simulink model "OM1"  (R2018b)
settings: Solver=VariableStepAuto  StartTime=0.0  StopTime=t_final  MaxStep=0.001  RelTol=1e-3
undefined symbols (not defined in the file): K1, K2, Ki, Kia, Kp, Kpa, st, T0, T1, T2, Tzap
settings Model: Creator=Anton Mayorov  LastModifiedBy=bedla
settings SFSimCC: SimUseLocalCustomCode=off
settings RTWCC: RTWUseLocalCustomCode=off

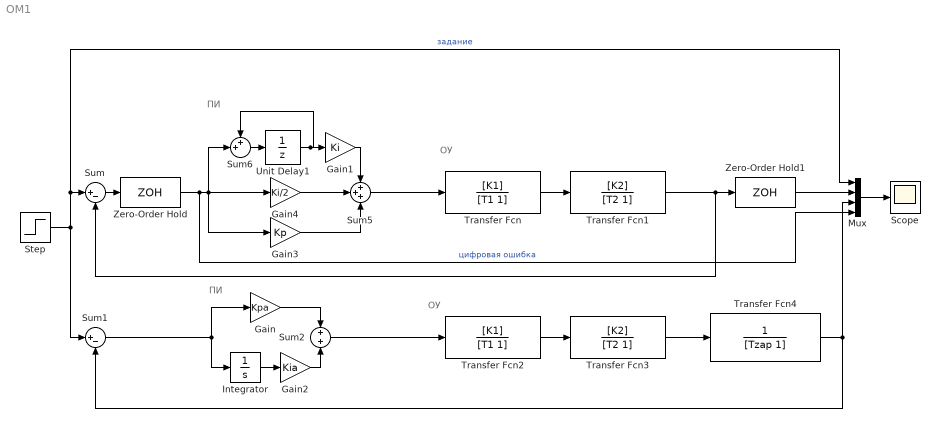
== system OM1 ==
  note: ПИ
  note: ПИ
  note: ОУ
  note: ОУ
  Gain : Gain  Gain=Kpa
  Gain1 : Gain  Gain=Ki
  Gain2 : Gain  Gain=Kia
  Gain3 : Gain  Gain=Kp
  Gain4 : Gain  Gain=Ki/2
  Integrator : Integrator
  Mux : Mux
  Scope : Scope
  Step : Step  Time=st  SampleTime=0
  Sum : Sum  Inputs=|+-
  Sum1 : Sum  Inputs=|+-
  Sum2 : Sum
  Sum5 : Sum  Inputs=+++
  Sum6 : Sum  Inputs=++|
  Transfer Fcn : TransferFcn  Numerator=[K1]  Denominator=[T1 1]
  Transfer Fcn1 : TransferFcn  Numerator=[K2]  Denominator=[T2 1]
  Transfer Fcn2 : TransferFcn  Numerator=[K1]  Denominator=[T1 1]
  Transfer Fcn3 : TransferFcn  Numerator=[K2]  Denominator=[T2 1]
  Transfer Fcn4 : TransferFcn  Denominator=[Tzap 1]
  Unit Delay1 : UnitDelay  SampleTime=-1  HasFrameUpgradeWarning=on
  Zero-Order Hold : ZeroOrderHold  SampleTime=T0
  Zero-Order Hold1 : ZeroOrderHold  SampleTime=T0
  wires:
  Gain/1 -> Sum2/1
  Gain2/1 -> Sum2/2
  Integrator/1 -> Gain2/1
  Sum5/1 -> Transfer Fcn/1
  Step/1 -> Mux/1, Sum/1, Sum1/1  "задание"
  Transfer Fcn/1 -> Transfer Fcn1/1
  Zero-Order Hold/1 -> Gain4/1, Gain3/1, Sum6/2, Mux/4  "цифровая ошибка"
  Transfer Fcn1/1 -> Sum/2, Zero-Order Hold1/1
  Sum6/1 -> Unit Delay1/1
  Sum/1 -> Zero-Order Hold/1
  Transfer Fcn4/1 -> Sum1/2, Mux/3
  Transfer Fcn2/1 -> Transfer Fcn3/1
  Transfer Fcn3/1 -> Transfer Fcn4/1
  Mux/1 -> Scope/1
  Zero-Order Hold1/1 -> Mux/2
  Gain4/1 -> Sum5/2
  Unit Delay1/1 -> Sum6/1, Gain1/1
  Gain3/1 -> Sum5/3
  Gain1/1 -> Sum5/1
  Sum1/1 -> Gain/1, Integrator/1
  Sum2/1 -> Transfer Fcn2/1
